simulink model "BATTERY"  (R2023b)
settings: Solver=VariableStepAuto  StartTime=0.0  StopTime=10.0  RelTol=1e-3
settings Model: Creator=lucaerviati  LastModifiedBy=carol
settings OptimizationCC: ReuseModelBlockBuffer=off

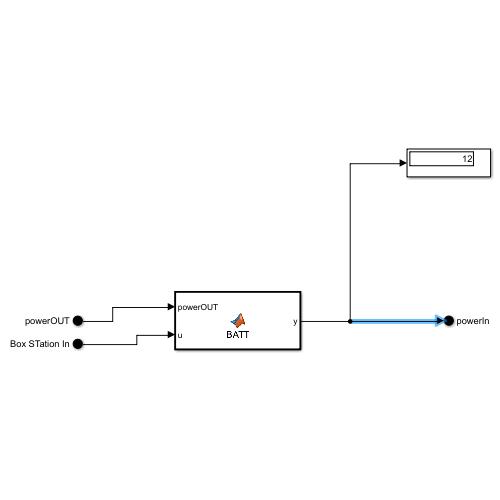
[thumbnail: Simulink's stored preview of the top-level diagram]
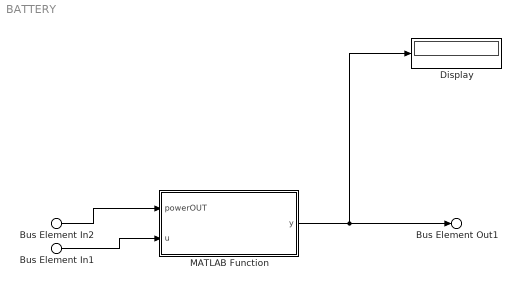
== system BATTERY ==
  Bus Element In2 : Inport  PortName=powerOUT
  Bus Element In1 : Inport  Port=2  PortName=Box STation In
  Display : Display
  MATLAB Function : MATLAB Function  TreatAsAtomicUnit=on
  Bus Element Out1 : Outport  PortName=powerIn
  wires:
  Bus Element In1/1 -> MATLAB Function/2(u)
  Bus Element In2/1 -> MATLAB Function/1(powerOUT)
  MATLAB Function/1(y) -> Bus Element Out1/1, Display/1

== matlab function BATTERY/MATLAB Function ==
  data: powerOUT input; u input; y output
function y = BATT(powerOUT, u)
u = 12
y = u;
